simulink model "Final_Version"  (R2016a)
settings: Solver=VariableStepAuto  StartTime=0.0  StopTime=500  FixedStep=0.0001  RelTol=1e-3
libraries: powerlib x5
settings Model: Creator=Seo  LastModifiedBy=Seo
settings DebuggingCC: MaxConsecutiveZCsMsg=none

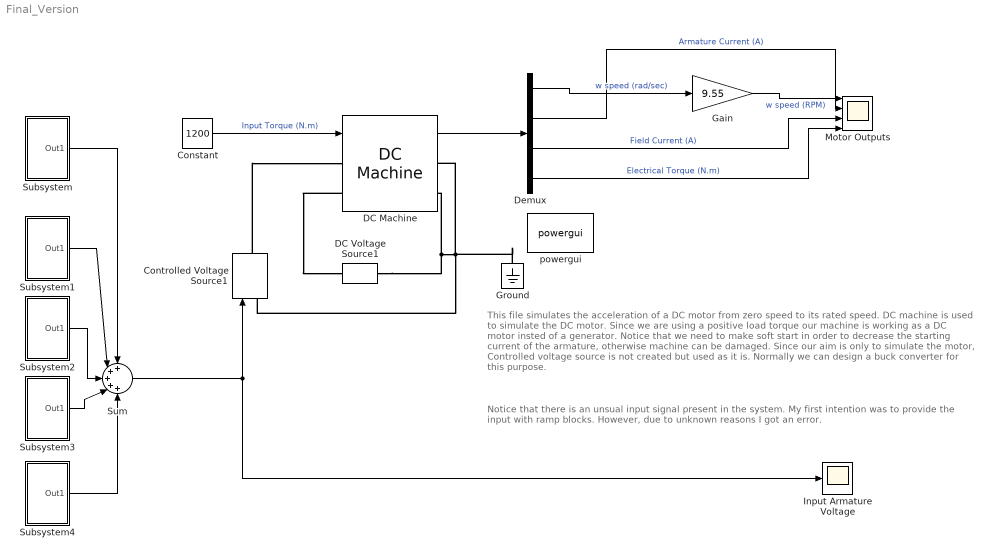
== system Final_Version ==
  note: Notice that there is  an unsual input signal present in the system. My first intention was  to provide the input
      | with ramp blocks. However, due to unknown reasons I got an error.
  note: This file simulates the acceleration of a DC motor from zero speed to its  rated speed.
      | DC machine is used to simulate the DC motor. Since we are using a positive load torque
      | our machine is working as a DC motor insted of a generator. Notice that we need to make
      | soft start in order to decrease the starting current of the armature, otherwise machine can be damaged.
      | Since our aim is only to simulate the motor, Controlled voltage source is not created but used as it is. Normally
      | we can design a buck converter for this purpose.
  Constant : Constant  Value=1200
  Controlled Voltage Source1 : powerlib/Electrical Sources/Controlled Voltage Source  Initialize=on  Source_Type=DC  Amplitude=0  Phase=0  Frequency=0  Measurements=None
  DC Machine : powerlib/Machines/DC Machine  PresetModel=18: 175HP 500V 1750RPM Field:300V  MechanicalLoad=Torque TL  FieldType=Wound  ShowDetailedParameters=on  MeasurementBus=off  RLa=[0.1009 0.002293]  RLf=[40.36 4.396]  Laf=0.3459  MachineConstant=Torque constant (N.m/A)  Ke=1.8  Kt=1.8  J=0.7142  Bm=0.01836  Tf=18.52  w0=1  Ifinit=1  TsPowergui=0  TsBlock=-1
  DC Voltage Source1 : powerlib/Electrical Sources/DC Voltage Source  Amplitude=300  Measurements=None
  Demux : Demux
  Gain : Gain  Gain=9.55
  Ground : powerlib/Elements/Ground  LConnTagsString=a
  Input Armature Voltage : Scope
  Motor Outputs : Scope  NumInputPorts=4
  Subsystem : Subsystem
  Subsystem1 : Subsystem
  Subsystem2 : Subsystem
  Subsystem3 : Subsystem
  Subsystem4 : Subsystem
  Sum : Sum  Inputs=+++++
  powergui : powerlib/powergui  Priority=1  SimulationMode=Continuous  SolverType=Tustin/Backward Euler (TBE)  SampleTime=50e-6  frequency=60  SPID=off  DisableSnubberDevices=off  DisableRonSwitches=off  DisableVfSwitches=off  SwTol=0  DisplayEquations=off  Interpol=off  ExternalGateDelay=off  methode=off  Ts=10  FunctionMessages=off  echomessages=off  HookPort=off  EnableUseOfTLC=off  x0status=blocks  frequencyindice=0  Pbase=100e6  ErrMax=1e-4  Iterations=50  UnitsV=kV  UnitsW=MW  buscounter=0  RestoreLinks=warning  ResistiveCurrentMeasurement=off  Frange=[0:2:500]  Ylog=off  Xlog=on  ShowGrid=off  save=off  variable=ZData  structure=0  ZoomFFT=off  StartTime=0.0  cycles=1  DisplayStyle=1  fundamental=60  FreqAxis=off  MaxFrequency=1000  frequencyindicesteady=1  RmsSteady=1  display=off
  wires:
  DC Machine/1 -> Demux/1
  Demux/1 -> Gain/1  "w speed (rad/sec)"
  Demux/2 -> Motor Outputs/2  "Armature Current (A)"
  Demux/3 -> Motor Outputs/3  "Field Current (A)"
  Demux/4 -> Motor Outputs/4  "Electrical Torque (N.m)"
  Constant/1 -> DC Machine/1  "Input Torque (N.m)"
  Gain/1 -> Motor Outputs/1  "w speed (RPM)"
  Sum/1 -> Input Armature Voltage/1, Controlled Voltage Source1/1
  Subsystem4/1(Out1) -> Sum/5
  Subsystem3/1(Out1) -> Sum/4
  Subsystem2/1(Out1) -> Sum/3
  Subsystem1/1(Out1) -> Sum/2
  Subsystem/1(Out1) -> Sum/1
  connections:
  DC Machine/LConn2 -- DC Voltage Source1/RConn1
  DC Voltage Source1/LConn1 -- Controlled Voltage Source1/LConn1 -- DC Machine/RConn1 -- Ground/LConn1 -- DC Machine/RConn2
  Controlled Voltage Source1/RConn1 -- DC Machine/LConn1

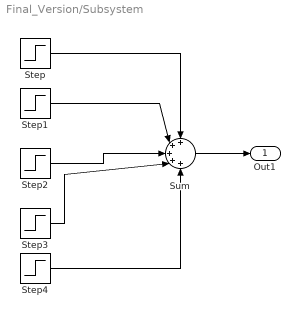
== system Final_Version/Subsystem ==
  Step : Step  After=20  SampleTime=0
  Step1 : Step  Time=10  After=20  SampleTime=0
  Step2 : Step  Time=20  After=20  SampleTime=0
  Step3 : Step  Time=30  After=20  SampleTime=0
  Step4 : Step  Time=40  After=20  SampleTime=0
  Sum : Sum  Inputs=+++++
  Out1 : Outport
  wires:
  Step/1 -> Sum/1
  Step3/1 -> Sum/4
  Sum/1 -> Out1/1
  Step2/1 -> Sum/3
  Step1/1 -> Sum/2
  Step4/1 -> Sum/5

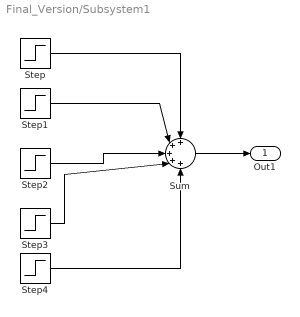
== system Final_Version/Subsystem1 ==
  Step : Step  Time=60  After=20  SampleTime=0
  Step1 : Step  Time=70  After=20  SampleTime=0
  Step2 : Step  Time=80  After=20  SampleTime=0
  Step3 : Step  Time=90  After=20  SampleTime=0
  Step4 : Step  Time=100  After=20  SampleTime=0
  Sum : Sum  Inputs=+++++
  Out1 : Outport
  wires:
  Step/1 -> Sum/1
  Step3/1 -> Sum/4
  Sum/1 -> Out1/1
  Step2/1 -> Sum/3
  Step1/1 -> Sum/2
  Step4/1 -> Sum/5

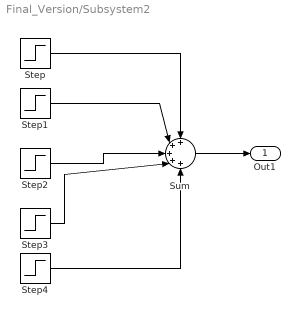
== system Final_Version/Subsystem2 ==
  Step : Step  Time=110  After=20  SampleTime=0
  Step1 : Step  Time=120  After=20  SampleTime=0
  Step2 : Step  Time=130  After=20  SampleTime=0
  Step3 : Step  Time=140  After=20  SampleTime=0
  Step4 : Step  Time=150  After=20  SampleTime=0
  Sum : Sum  Inputs=+++++
  Out1 : Outport
  wires:
  Step/1 -> Sum/1
  Step3/1 -> Sum/4
  Sum/1 -> Out1/1
  Step2/1 -> Sum/3
  Step1/1 -> Sum/2
  Step4/1 -> Sum/5

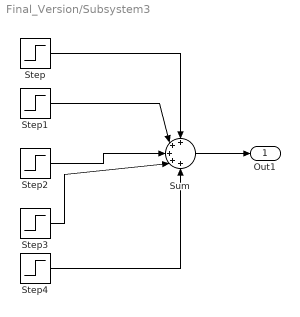
== system Final_Version/Subsystem3 ==
  Step : Step  Time=160  After=20  SampleTime=0
  Step1 : Step  Time=170  After=20  SampleTime=0
  Step2 : Step  Time=180  After=20  SampleTime=0
  Step3 : Step  Time=190  After=20  SampleTime=0
  Step4 : Step  Time=200  After=20  SampleTime=0
  Sum : Sum  Inputs=+++++
  Out1 : Outport
  wires:
  Step/1 -> Sum/1
  Step3/1 -> Sum/4
  Sum/1 -> Out1/1
  Step2/1 -> Sum/3
  Step1/1 -> Sum/2
  Step4/1 -> Sum/5

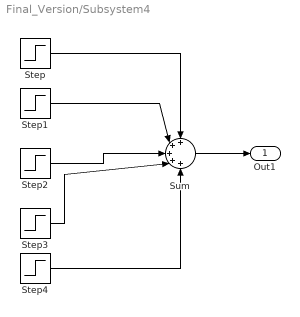
== system Final_Version/Subsystem4 ==
  Step : Step  Time=210  After=20  SampleTime=0
  Step1 : Step  Time=220  After=20  SampleTime=0
  Step2 : Step  Time=230  After=20  SampleTime=0
  Step3 : Step  Time=240  After=20  SampleTime=0
  Step4 : Step  Time=250  After=20  SampleTime=0
  Sum : Sum  Inputs=+++++
  Out1 : Outport
  wires:
  Step/1 -> Sum/1
  Step3/1 -> Sum/4
  Sum/1 -> Out1/1
  Step2/1 -> Sum/3
  Step1/1 -> Sum/2
  Step4/1 -> Sum/5
